simulink model "ROS2_simulink_UE5_0821"  (R2024b)
settings: Solver=VariableStepAuto  StartTime=0.0  StopTime=inf  RelTol=1e-3
undefined symbols (not defined in the file): Aw_pont, B_pont, Cb_pont, dt, Earth, I_L, I_T, IC, Ig_CG, k_neg, k_pos, L, l1, l2, LCF, m, rg, Sim3dSensor, T_yaw, trim_setpoint, Umax, WGS84, x, y, z
libraries: sim3dlib x12, ros2lib x8, matrix_library x8, sharedutil x7, uavsimlib x6, simulink x4, simulink_extras x4, sharedtransform x3, robotcorelib x1, aerolibtransform2 x1, sim3dcameralib x1, visionsinks x1
(part 2 of 2)

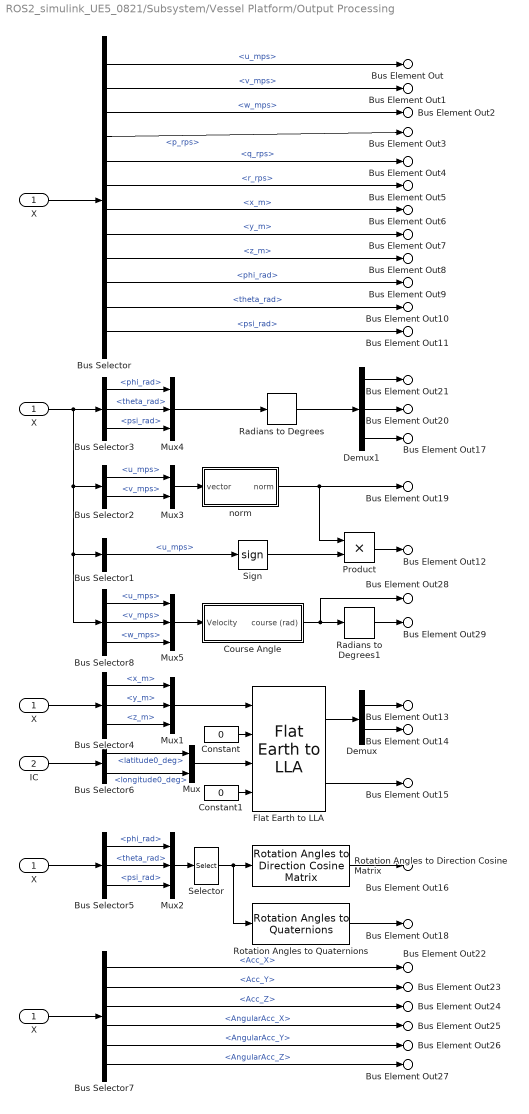
== system ROS2_simulink_UE5_0821/Subsystem/Vessel Platform/Output Processing ==
  X : Inport
  IC : Inport  Port=2
  " X" : InportShadow
  " X  " : InportShadow
  Bus Selector : BusSelector  OutputSignals=u_mps,v_mps,w_mps,p_rps,q_rps,r_rps,x_m,y_m,z_m,phi_rad,theta_rad,psi_rad
  Bus Selector1 : BusSelector  OutputSignals=u_mps
  Bus Selector2 : BusSelector  OutputSignals=u_mps,v_mps
  Bus Selector3 : BusSelector  OutputSignals=phi_rad,theta_rad,psi_rad
  Bus Selector4 : BusSelector  OutputSignals=x_m,y_m,z_m
  Bus Selector5 : BusSelector  OutputSignals=phi_rad,theta_rad,psi_rad
  Bus Selector6 : BusSelector  OutputSignals=latitude0_deg,longitude0_deg
  Bus Selector7 : BusSelector  OutputSignals=Acc_X,Acc_Y,Acc_Z,AngularAcc_X,AngularAcc_Y,AngularAcc_Z
  Bus Selector8 : BusSelector  OutputSignals=u_mps,v_mps,w_mps
  Constant : Constant  Value=0
  Constant1 : Constant  Value=0
  Course Angle : Subsystem
  Demux : Demux  Outputs=2
  Demux1 : Demux  Outputs=3
  Flat Earth to LLA : aerolibtransform2/Flat Earth to LLA  units=Metric (MKS)  ptype=Earth (WGS84)  F=1/298.257223563  R=6378137  refPosPort=on  LL0=ll0  psi=0
  Mux : Mux  Inputs=2
  Mux{1..2,4..5} (4 alike) : Mux  Inputs=3
  Mux3 : Mux  Inputs=2
  Product : Product
  Radians to Degrees : simulink_extras/Transformations/Radians to Degrees
  Radians to Degrees1 : simulink_extras/Transformations/Radians to Degrees
  Rotation Angles to Direction Cosine Matrix : sharedtransform/Rotation Angles to Direction Cosine Matrix  rotationOrder=ZYX  aMode=aMode
  Rotation Angles to Quaternions : sharedtransform/Rotation Angles to Quaternions  rotationOrder=ZYX  aMode=aMode
  Selector : Selector  InputPortWidth=3  IndexOptions=Index vector (dialog)  Indices=[3 2 1]  OutputSizes=1
  Sign : Signum
  "X " : InportShadow
  "X  " : InportShadow
  norm : Subsystem
  Bus Element Out : Outport  PortName=VesselStates  Element=Surge Velocity (m/s)
  Bus Element Out1 : Outport  PortName=VesselStates  Element=Sway Velocity (m/s)
  Bus Element Out2 : Outport  PortName=VesselStates  Element=Heave Velocity (m/s)
  Bus Element Out3 : Outport  PortName=VesselStates  Element=Roll Rate (rad/s)
  Bus Element Out4 : Outport  PortName=VesselStates  Element=Pitch Rate (rad/s)
  Bus Element Out5 : Outport  PortName=VesselStates  Element=Yaw Rate (rad/s)
  Bus Element Out6 : Outport  PortName=VesselStates  Element=x (m)
  Bus Element Out7 : Outport  PortName=VesselStates  Element=y (m)
  Bus Element Out8 : Outport  PortName=VesselStates  Element=z (m)
  Bus Element Out9 : Outport  PortName=VesselStates  Element=Roll Angle (rad)
  Bus Element Out10 : Outport  PortName=VesselStates  Element=Pitch Angle (rad)
  Bus Element Out11 : Outport  PortName=VesselStates  Element=Yaw Angle (rad)
  Bus Element Out21 : Outport  PortName=VesselStates  Element=Roll Angle (deg)
  Bus Element Out20 : Outport  PortName=VesselStates  Element=Pitch Angle (deg)
  Bus Element Out17 : Outport  PortName=VesselStates  Element=Yaw Angle (deg)
  Bus Element Out12 : Outport  PortName=VesselStates  Element=speed (signed m/s)
  Bus Element Out19 : Outport  PortName=VesselStates  Element=speed (unsigned m/s)
  Bus Element Out13 : Outport  PortName=VesselStates  Element=latitude (deg)
  Bus Element Out14 : Outport  PortName=VesselStates  Element=longitude (deg)
  Bus Element Out15 : Outport  PortName=VesselStates  Element=altitude (m)
  Bus Element Out16 : Outport  PortName=VesselStates  Element=DCM_be
  Bus Element Out18 : Outport  PortName=VesselStates  Element=Quaternion
  Bus Element Out22 : Outport  PortName=VesselStates  Element=Acc X (m/s2)
  Bus Element Out23 : Outport  PortName=VesselStates  Element=Acc Y (m/s2)
  Bus Element Out24 : Outport  PortName=VesselStates  Element=Acc Z (m/s2)
  Bus Element Out25 : Outport  PortName=VesselStates  Element=Angular Acc X (rad/s2)
  Bus Element Out26 : Outport  PortName=VesselStates  Element=Angular Acc Y (rad/s2)
  Bus Element Out27 : Outport  PortName=VesselStates  Element=Angular Acc Z (rad/s2)
  Bus Element Out28 : Outport  PortName=VesselStates  Element=course (rad)
  Bus Element Out29 : Outport  PortName=VesselStates  Element=course (deg)
  wires:
  Demux/1 -> Bus Element Out13/1
  Rotation Angles to Quaternions/1 -> Bus Element Out18/1
  Product/1 -> Bus Element Out12/1
  Rotation Angles to Direction Cosine Matrix/1 -> Bus Element Out16/1
  Demux/2 -> Bus Element Out14/1
  Constant/1 -> Flat Earth to LLA/2
  Mux1/1 -> Flat Earth to LLA/1
  Flat Earth to LLA/1 -> Demux/1
  Flat Earth to LLA/2 -> Bus Element Out15/1
  X/1 -> Bus Selector/1
  Bus Selector/1 -> Bus Element Out/1  "<u_mps>"
  Bus Selector/2 -> Bus Element Out1/1  "<v_mps>"
  Bus Selector/3 -> Bus Element Out2/1  "<w_mps>"
  Bus Selector/4 -> Bus Element Out3/1  "<p_rps>"
  Bus Selector/5 -> Bus Element Out4/1  "<q_rps>"
  Bus Selector/6 -> Bus Element Out5/1  "<r_rps>"
  Bus Selector/7 -> Bus Element Out6/1  "<x_m>"
  Bus Selector/8 -> Bus Element Out7/1  "<y_m>"
  Bus Selector/9 -> Bus Element Out8/1  "<z_m>"
  Bus Selector/10 -> Bus Element Out9/1  "<phi_rad>"
  Bus Selector/11 -> Bus Element Out10/1  "<theta_rad>"
  Bus Selector/12 -> Bus Element Out11/1  "<psi_rad>"
  Bus Selector1/1 -> Sign/1  "<u_mps>"
  "X "/1 -> Bus Selector8/1, Bus Selector1/1, Bus Selector2/1, Bus Selector3/1
  Mux3/1 -> norm/1(vector)
  Bus Selector2/1 -> Mux3/1  "<u_mps>"
  Bus Selector2/2 -> Mux3/2  "<v_mps>"
  norm/1(norm) -> Product/1, Bus Element Out19/1
  Bus Selector4/1 -> Mux1/1  "<x_m>"
  Bus Selector4/2 -> Mux1/2  "<y_m>"
  Bus Selector4/3 -> Mux1/3  "<z_m>"
  IC/1 -> Bus Selector6/1
  Bus Selector6/1 -> Mux/1  "<latitude0_deg>"
  Bus Selector6/2 -> Mux/2  "<longitude0_deg>"
  Mux/1 -> Flat Earth to LLA/3
  Selector/1 -> Rotation Angles to Quaternions/1, Rotation Angles to Direction Cosine Matrix/1
  Bus Selector5/1 -> Mux2/1  "<phi_rad>"
  Bus Selector5/2 -> Mux2/2  "<theta_rad>"
  Bus Selector5/3 -> Mux2/3  "<psi_rad>"
  Mux2/1 -> Selector/1
  "X  "/1 -> Bus Selector4/1
  " X"/1 -> Bus Selector5/1
  Bus Selector3/1 -> Mux4/1  "<phi_rad>"
  Bus Selector3/2 -> Mux4/2  "<theta_rad>"
  Bus Selector3/3 -> Mux4/3  "<psi_rad>"
  Mux4/1 -> Radians to Degrees/1
  Radians to Degrees/1 -> Demux1/1
  Demux1/3 -> Bus Element Out17/1
  Demux1/2 -> Bus Element Out20/1
  Demux1/1 -> Bus Element Out21/1
  " X  "/1 -> Bus Selector7/1
  Bus Selector7/1 -> Bus Element Out22/1  "<Acc_X>"
  Bus Selector7/2 -> Bus Element Out23/1  "<Acc_Y>"
  Bus Selector7/3 -> Bus Element Out24/1  "<Acc_Z>"
  Bus Selector7/4 -> Bus Element Out25/1  "<AngularAcc_X>"
  Bus Selector7/5 -> Bus Element Out26/1  "<AngularAcc_Y>"
  Bus Selector7/6 -> Bus Element Out27/1  "<AngularAcc_Z>"
  Constant1/1 -> Flat Earth to LLA/4
  Sign/1 -> Product/2
  Bus Selector8/3 -> Mux5/3  "<w_mps>"
  Bus Selector8/2 -> Mux5/2  "<v_mps>"
  Bus Selector8/1 -> Mux5/1  "<u_mps>"
  Mux5/1 -> Course Angle/1(Velocity)
  Course Angle/1(course (rad)) -> Bus Element Out28/1, Radians to Degrees1/1
  Radians to Degrees1/1 -> Bus Element Out29/1

== system ROS2_simulink_UE5_0821/Subsystem/Vessel Platform/Sum of Forces and Moments ==
  Thrust : Inport
  Crossflow : Inport  Port=2
  Bus Element In7 : Inport  Port=3  PortName=Hydrodynamics  Element=Coriolis
  Bus Element In1 : Inport  Port=3  PortName=Hydrodynamics  Element=Damping
  Bus Element In6 : Inport  Port=4  PortName=Hydrostatic  Element=Hydrostatic
  Bus Element In2 : Inport  Port=4  PortName=Hydrostatic  Element=Ballast
  Add : Sum  Inputs=+++---
  Bus Creator : BusCreator  Inputs=1
  Forces and Moments : Outport
  wires:
  Crossflow/1 -> Add/3
  Bus Element In1/1 -> Add/2
  Bus Element In7/1 -> Add/4
  Thrust/1 -> Add/1
  Add/1 -> Bus Creator/1  "force_moment"
  Bus Creator/1 -> Forces and Moments/1
  Bus Element In6/1 -> Add/5
  Bus Element In2/1 -> Add/6

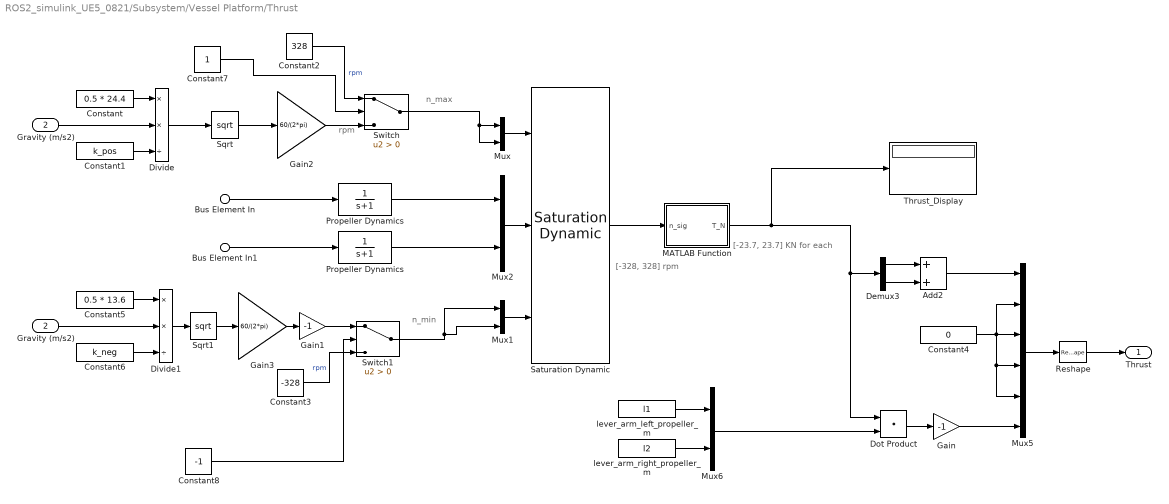
== system ROS2_simulink_UE5_0821/Subsystem/Vessel Platform/Thrust ==
  note: rpm
  note: n_max
  note: n_min
  note: [-23.7, 23.7] KN for each
  note: [-328, 328] rpm
  Bus Element In : Inport  PortName=VesselCmds  Element=PropellerCommand_L_rpm
  Bus Element In1 : Inport  PortName=VesselCmds  Element=PropellerCommand_R_rpm
  "Gravity (m/s2) " : Inport  Port=2
  Add2 : Sum
  Constant : Constant  Value=0.5 * 24.4
  Constant1 : Constant  Value=k_pos
  Constant2 : Constant  Value=328
  Constant3 : Constant  Value=-328
  Constant4 : Constant  Value=0
  Constant5 : Constant  Value=0.5 * 13.6
  Constant6 : Constant  Value=k_neg
  Constant7 : Constant
  Constant8 : Constant  Value=-1
  Demux3 : Demux  Outputs=2
  Divide : Product  Inputs=**/
  Divide1 : Product  Inputs=**/
  Dot Product : DotProduct  OutDataTypeStr=Inherit: Inherit via internal rule
  Gain : Gain  Gain=-1
  Gain1 : Gain  Gain=-1
  Gain2 : Gain  Gain=60/(2*pi)
  Gain3 : Gain  Gain=60/(2*pi)
  "Gravity (m/s2)  " : InportShadow  Port=2
  MATLAB Function : MATLAB Function  TreatAsAtomicUnit=on
  Mux{,1..2,6} (4 alike) : Mux  Inputs=2
  Mux5 : Mux  Inputs=6
  Propeller Dynamics : TransferFcn  Denominator=[1 1]
  "Propeller Dynamics " : TransferFcn  Denominator=[1 1]
  Reshape : Reshape  OutputDimensionality=Column vector (2-D)
  Saturation Dynamic : simulink/Discontinuities/Saturation Dynamic  OutMin=[]  OutMax=[]  OutDataTypeStr=Inherit: Same as second input  OutDataType=fixdt(1, 16)  OutScaling=2^-10  DoSatur=off
  Sqrt : Sqrt
  Sqrt1 : Sqrt
  Switch : Switch  Criteria=u2 > Threshold  SaturateOnIntegerOverflow=off  InputSameDT=off
  Switch1 : Switch  Criteria=u2 > Threshold  SaturateOnIntegerOverflow=off  InputSameDT=off
  Thrust_Display : Display
  lever_arm_left_propeller_m : Constant  Value=l1
  lever_arm_right_propeller_m : Constant  Value=l2
  Thrust : Outport
  wires:
  Saturation Dynamic/1 -> MATLAB Function/1(n_sig)
  Demux3/2 -> Add2/2
  Dot Product/1 -> Gain/1
  Gain/1 -> Mux5/6
  Mux5/1 -> Reshape/1
  Mux6/1 -> Dot Product/2
  Add2/1 -> Mux5/1
  Constant4/1 -> Mux5/5, Mux5/4, Mux5/2, Mux5/3
  Demux3/1 -> Add2/1
  lever_arm_right_propeller_m/1 -> Mux6/2
  lever_arm_left_propeller_m/1 -> Mux6/1
  Reshape/1 -> Thrust/1
  Constant/1 -> Divide/1
  "Gravity (m/s2) "/1 -> Divide/2
  Constant1/1 -> Divide/3
  Divide/1 -> Sqrt/1
  Divide1/1 -> Sqrt1/1
  Constant5/1 -> Divide1/1
  "Gravity (m/s2)  "/1 -> Divide1/2
  Constant6/1 -> Divide1/3
  Sqrt1/1 -> Gain3/1
  Mux/1 -> Saturation Dynamic/1
  Sqrt/1 -> Gain2/1
  Mux1/1 -> Saturation Dynamic/3
  Mux2/1 -> Saturation Dynamic/2
  Bus Element In/1 -> Propeller Dynamics/1
  Bus Element In1/1 -> "Propeller Dynamics "/1
  "Propeller Dynamics "/1 -> Mux2/2
  Gain2/1 -> Switch/3
  MATLAB Function/1(T_N) -> Thrust_Display/1, Dot Product/1, Demux3/1
  Propeller Dynamics/1 -> Mux2/1
  Switch/1 -> Mux/1, Mux/2
  Constant2/1 -> Switch/1  "rpm"
  Gain3/1 -> Gain1/1
  Gain1/1 -> Switch1/1
  Switch1/1 -> Mux1/2, Mux1/1
  Constant3/1 -> Switch1/3  "rpm"
  Constant7/1 -> Switch/2
  Constant8/1 -> Switch1/2

== system ROS2_simulink_UE5_0821/Subsystem/Vessel Platform/Waves and Crossflow ==
  RelativeVelocity : Inport
  Draft (m) : Inport  Port=2
  "Water Density (kg/m3) " : Inport  Port=3
  Compute tau_crossflow : MATLAB Function  TreatAsAtomicUnit=on
  beam_pontoon_m : Constant  Value=B_pont
  length_m : Constant  Value=L
  Crossflow : Outport
  wires:
  length_m/1 -> Compute tau_crossflow/1(L)
  RelativeVelocity/1 -> Compute tau_crossflow/4(nu_r)
  Compute tau_crossflow/1(tau_crossflow) -> Crossflow/1
  beam_pontoon_m/1 -> Compute tau_crossflow/2(B)
  "Water Density (kg/m3) "/1 -> Compute tau_crossflow/5(rho)
  Draft (m)/1 -> Compute tau_crossflow/3(T)

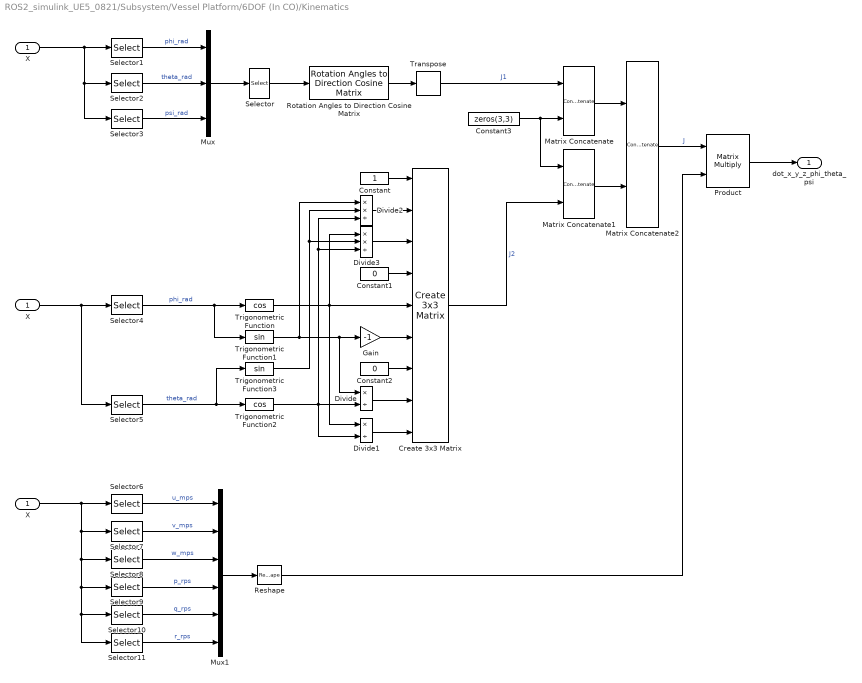
== system ROS2_simulink_UE5_0821/Subsystem/Vessel Platform/6DOF (In CO)/Kinematics ==
  X : Inport
  Constant : Constant
  Constant1 : Constant  Value=0
  Constant2 : Constant  Value=0
  Constant3 : Constant  Value=zeros(3,3)
  Create 3x3 Matrix : sharedutil/Create 3x3 Matrix  aMode=aMode
  Divide : Product  Inputs=*/
  Divide1 : Product  Inputs=*/
  Divide2 : Product  Inputs=**/
  Divide3 : Product  Inputs=**/
  Gain : Gain  Gain=-1
  Matrix Concatenate : Concatenate  Mode=Multidimensional array  ConcatenateDimension=2
  Matrix Concatenate1 : Concatenate  Mode=Multidimensional array  ConcatenateDimension=2
  Matrix Concatenate2 : Concatenate  Mode=Multidimensional array
  Mux : Mux  Inputs=3
  Mux1 : Mux  Inputs=6
  Product : Product  Multiplication=Matrix(*)
  Reshape : Reshape  OutputDimensionality=Column vector (2-D)
  Rotation Angles to Direction Cosine Matrix : sharedtransform/Rotation Angles to Direction Cosine Matrix  rotationOrder=ZYX  aMode=aMode
  Selector : Selector  InputPortWidth=3  IndexOptions=Index vector (dialog)  Indices=[3 2 1]  OutputSizes=1
  Selector1 : Selector  InputPortWidth=12  IndexOptions=Index vector (dialog)  Indices=[10]  OutputSizes=1
  Selector10 : Selector  InputPortWidth=12  IndexOptions=Index vector (dialog)  Indices=[5]  OutputSizes=1
  Selector11 : Selector  InputPortWidth=12  IndexOptions=Index vector (dialog)  Indices=[6]  OutputSizes=1
  Selector2 : Selector  InputPortWidth=12  IndexOptions=Index vector (dialog)  Indices=[11]  OutputSizes=1
  Selector3 : Selector  InputPortWidth=12  IndexOptions=Index vector (dialog)  Indices=[12]  OutputSizes=1
  Selector4 : Selector  InputPortWidth=12  IndexOptions=Index vector (dialog)  Indices=[10]  OutputSizes=1
  Selector5 : Selector  InputPortWidth=12  IndexOptions=Index vector (dialog)  Indices=[11]  OutputSizes=1
  Selector6 : Selector  InputPortWidth=12  IndexOptions=Index vector (dialog)  Indices=[1]  OutputSizes=1
  Selector7 : Selector  InputPortWidth=12  IndexOptions=Index vector (dialog)  Indices=[2]  OutputSizes=1
  Selector8 : Selector  InputPortWidth=12  IndexOptions=Index vector (dialog)  Indices=[3]  OutputSizes=1
  Selector9 : Selector  InputPortWidth=12  IndexOptions=Index vector (dialog)  Indices=[4]  OutputSizes=1
  Transpose : matrix_library/Transpose
  Trigonometric Function : Trigonometry  Operator=cos
  Trigonometric Function1 : Trigonometry
  Trigonometric Function2 : Trigonometry  Operator=cos
  Trigonometric Function3 : Trigonometry
  "X " : InportShadow
  "X  " : InportShadow
  dot_x_y_z_phi_theta_psi : Outport
  wires:
  Rotation Angles to Direction Cosine Matrix/1 -> Transpose/1
  Selector/1 -> Rotation Angles to Direction Cosine Matrix/1
  Selector1/1 -> Mux/1  "phi_rad"
  Selector2/1 -> Mux/2  "theta_rad"
  Selector3/1 -> Mux/3  "psi_rad"
  Mux/1 -> Selector/1
  Constant/1 -> Create 3x3 Matrix/1
  Constant1/1 -> Create 3x3 Matrix/4
  Constant2/1 -> Create 3x3 Matrix/7
  Trigonometric Function/1 -> Divide3/1, Divide1/1, Create 3x3 Matrix/5
  Selector4/1 -> Trigonometric Function1/1, Trigonometric Function/1  "phi_rad"
  Trigonometric Function1/1 -> Divide/1, Gain/1, Divide2/1
  Gain/1 -> Create 3x3 Matrix/6
  Selector5/1 -> Trigonometric Function3/1, Trigonometric Function2/1  "theta_rad"
  Divide/1 -> Create 3x3 Matrix/8
  Trigonometric Function2/1 -> Divide3/3, Divide2/3, Divide1/2, Divide/2
  Divide1/1 -> Create 3x3 Matrix/9
  Divide2/1 -> Create 3x3 Matrix/2
  Divide3/1 -> Create 3x3 Matrix/3
  Trigonometric Function3/1 -> Divide3/2, Divide2/2
  Matrix Concatenate/1 -> Matrix Concatenate2/1
  Matrix Concatenate1/1 -> Matrix Concatenate2/2
  Transpose/1 -> Matrix Concatenate/1  "J1"
  Constant3/1 -> Matrix Concatenate/2, Matrix Concatenate1/1
  Create 3x3 Matrix/1 -> Matrix Concatenate1/2  "J2"
  Selector6/1 -> Mux1/1  "u_mps"
  Selector7/1 -> Mux1/2  "v_mps"
  Selector8/1 -> Mux1/3  "w_mps"
  Selector9/1 -> Mux1/4  "p_rps"
  Selector10/1 -> Mux1/5  "q_rps"
  Selector11/1 -> Mux1/6  "r_rps"
  Mux1/1 -> Reshape/1
  X/1 -> Selector3/1, Selector2/1, Selector1/1
  "X "/1 -> Selector5/1, Selector4/1
  "X  "/1 -> Selector7/1, Selector8/1, Selector9/1, Selector10/1, Selector11/1, Selector6/1
  Matrix Concatenate2/1 -> Product/1  "J"
  Reshape/1 -> Product/2
  Product/1 -> dot_x_y_z_phi_theta_psi/1

== system ROS2_simulink_UE5_0821/Subsystem/Vessel Platform/6DOF (In CO)/ssa    ==
  angle : Inport
  " " : Math  Operator=mod
  Constant : Constant  Value=2*pi
  Constant1 : Constant  Value=pi
  Sum : Sum  Inputs=++|
  Sum1 : Sum  Inputs=-+|
  angle_pipi : Outport
  wires:
  Sum/1 -> " "/1
  Constant1/1 -> Sum/1, Sum1/1
  " "/1 -> Sum1/2
  Sum1/1 -> angle_pipi/1
  Constant/1 -> " "/2
  angle/1 -> Sum/2

== system ROS2_simulink_UE5_0821/Subsystem/Vessel Platform/Hydrodynamics/Coriolis  ==
  Relative Velocity : Inport
  Transform CG to CO : Inport  Port=2
  Inertial Matrix (hull and payload) in CO : Inport  Port=3
  X : Inport  Port=4
  Added Mass (Hydrodynamics) : Inport  Port=5
  Inertials : Inport  Port=6
  Bus Selector : BusSelector  OutputSignals=p_rps,q_rps,r_rps
  Bus Selector1 : BusSelector  OutputSignals=mp
  Compute CA : MATLAB Function  TreatAsAtomicUnit=on
  Comupute CRB : Subsystem
  Mux : Mux  Inputs=3
  Product : Product  Multiplication=Matrix(*)
  "Relative Velocity " : InportShadow
  Reshape : Reshape  OutputDimensionality=Column vector (2-D)
  Sum : Sum  Inputs=+|+
  Coriolis : Outport
  wires:
  Comupute CRB/1(CRB) -> Sum/2  "CRB"
  Added Mass (Hydrodynamics)/1 -> Compute CA/1(MA)
  "Relative Velocity "/1 -> Reshape/1
  Sum/1 -> Product/1  "C"
  Compute CA/1(CA) -> Sum/1  "CA"
  Reshape/1 -> Product/2
  Product/1 -> Coriolis/1
  Relative Velocity/1 -> Compute CA/2(nu_r)
  Bus Selector/1 -> Mux/1  "<p_rps>"
  Bus Selector/2 -> Mux/2  "<q_rps>"
  Bus Selector/3 -> Mux/3  "<r_rps>"
  Mux/1 -> Comupute CRB/1(pqr)
  X/1 -> Bus Selector/1
  Transform CG to CO/1 -> Comupute CRB/2(H)
  Inertial Matrix (hull and payload) in CO/1 -> Comupute CRB/3(Ig)
  Inertials/1 -> Bus Selector1/1
  Bus Selector1/1 -> Comupute CRB/4(mp)  "<mp>"

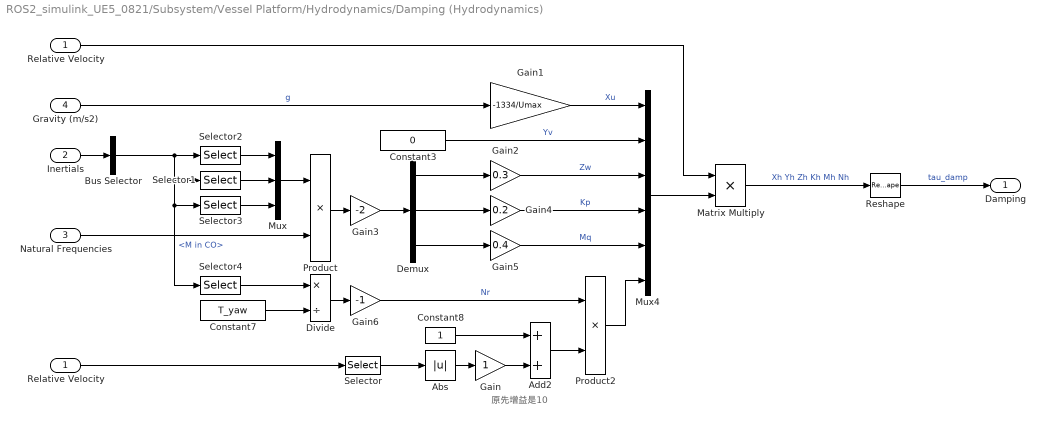
== system ROS2_simulink_UE5_0821/Subsystem/Vessel Platform/Hydrodynamics/Damping (Hydrodynamics) ==
  note: 原先增益是10
  Relative Velocity : Inport
  Inertials : Inport  Port=2
  Natural Frequencies : Inport  Port=3
  "Gravity (m/s2) " : Inport  Port=4
  Abs : Abs  SaturateOnIntegerOverflow=off
  Add2 : Sum
  Bus Selector : BusSelector  OutputSignals=M in CO
  Constant3 : Constant  Value=0
  Constant7 : Constant  Value=T_yaw
  Constant8 : Constant
  Demux : Demux  Outputs=3
  Divide : Product  Inputs=*/
  Gain : Gain
  Gain1 : Gain  Gain=-1334/Umax
  Gain2 : Gain  Gain=0.3
  Gain3 : Gain  Gain=-2
  Gain4 : Gain  Gain=0.2
  Gain5 : Gain  Gain=0.4
  Gain6 : Gain  Gain=-1
  Matrix Multiply : Product
  Mux : Mux  Inputs=3
  Mux4 : Mux  Inputs=6
  Product : Product
  Product2 : Product
  "Relative Velocity " : InportShadow
  Reshape : Reshape  OutputDimensionality=Column vector (2-D)
  Selector : Selector  InputPortWidth=6  IndexOptions=Index vector (dialog)  Indices=[6]  OutputSizes=1
  Selector1 : Selector  NumberOfDimensions=2  InputPortWidth=3  IndexOptions=Index vector (dialog),Index vector (dialog)  Indices=4,4  OutputSizes=1,1
  Selector2 : Selector  NumberOfDimensions=2  InputPortWidth=3  IndexOptions=Index vector (dialog),Index vector (dialog)  Indices=3,3  OutputSizes=1,1
  Selector3 : Selector  NumberOfDimensions=2  InputPortWidth=3  IndexOptions=Index vector (dialog),Index vector (dialog)  Indices=5,5  OutputSizes=1,1
  Selector4 : Selector  NumberOfDimensions=2  InputPortWidth=3  IndexOptions=Index vector (dialog),Index vector (dialog)  Indices=6,6  OutputSizes=1,1
  Damping : Outport
  wires:
  Constant3/1 -> Mux4/2  "Yv"
  Gain/1 -> Add2/2
  Gain1/1 -> Mux4/1  "Xu"
  Constant8/1 -> Add2/1
  Selector/1 -> Abs/1
  Demux/2 -> Gain4/1
  Gain6/1 -> Product2/1  "Nr"
  Product2/1 -> Mux4/6
  Abs/1 -> Gain/1
  Gain5/1 -> Mux4/5  "Mq"
  Gain2/1 -> Mux4/3  "Zw"
  Add2/1 -> Product2/2
  Mux4/1 -> Matrix Multiply/2
  Relative Velocity/1 -> Matrix Multiply/1
  Matrix Multiply/1 -> Reshape/1  "Xh Yh Zh Kh Mh Nh"
  Reshape/1 -> Damping/1  "tau_damp"
  "Gravity (m/s2) "/1 -> Gain1/1  "g"
  "Relative Velocity "/1 -> Selector/1
  Inertials/1 -> Bus Selector/1
  Bus Selector/1 -> Selector1/1, Selector4/1, Selector3/1, Selector2/1  "<M in CO>"
  Selector2/1 -> Mux/1
  Selector1/1 -> Mux/2
  Selector3/1 -> Mux/3
  Mux/1 -> Product/1
  Natural Frequencies/1 -> Product/2
  Product/1 -> Gain3/1
  Demux/1 -> Gain2/1
  Gain3/1 -> Demux/1
  Gain4/1 -> Mux4/4  "Kp"
  Demux/3 -> Gain5/1
  Selector4/1 -> Divide/1
  Constant7/1 -> Divide/2
  Divide/1 -> Gain6/1

== system ROS2_simulink_UE5_0821/Subsystem/Vessel Platform/Hydrostatic/Ballast ==
  Constant : Constant  Value=0
  Constant9 : Constant  Value=trim_setpoint
  Mux : Mux  Inputs=6
  Reshape : Reshape  OutputDimensionality=Column vector (2-D)
  Transfer Fcn2 : TransferFcn  Denominator=[1 1]
  Ballast : Outport
  wires:
  Constant9/1 -> Transfer Fcn2/1
  Transfer Fcn2/1 -> Mux/5
  Constant/1 -> Mux/2, Mux/3, Mux/6, Mux/4, Mux/1
  Mux/1 -> Reshape/1
  Reshape/1 -> Ballast/1

== system ROS2_simulink_UE5_0821/Subsystem/Vessel Platform/Input Processing/Added Mass (Hydrodynamics)  ==
  Inertial Matrix (hull and payload) in CO : Inport
  Create Diagonal Matrix : matrix_library/Create Diagonal Matrix
  Gain : Gain  Gain=-0.1
  Gain1 : Gain  Gain=-1
  Gain2 : Gain  Gain=-1.5
  Gain3 : Gain  Gain=-1
  Gain4 : Gain  Gain=-0.2
  Gain5 : Gain  Gain=-0.8
  Gain6 : Gain  Gain=-1.7
  Mux : Mux  Inputs=6
  Selector : Selector  NumberOfDimensions=2  InputPortWidth=3  IndexOptions=Index vector (dialog),Index vector (dialog)  Indices=1,1  OutputSizes=1,1
  Selector1 : Selector  NumberOfDimensions=2  InputPortWidth=3  IndexOptions=Index vector (dialog),Index vector (dialog)  Indices=2,2  OutputSizes=1,1
  Selector2 : Selector  NumberOfDimensions=2  InputPortWidth=3  IndexOptions=Index vector (dialog),Index vector (dialog)  Indices=3,3  OutputSizes=1,1
  "mass (kg) " : Constant  Value=m
  Added Mass (Hydrodynamcis) : Outport
  wires:
  Gain1/1 -> Added Mass (Hydrodynamcis)/1
  "mass (kg) "/1 -> Gain3/1, Gain2/1, Gain/1
  Create Diagonal Matrix/1 -> Gain1/1
  Mux/1 -> Create Diagonal Matrix/1
  Gain/1 -> Mux/1  "Xudot"
  Gain2/1 -> Mux/2  "Yvdot"
  Gain3/1 -> Mux/3  "Zwdot"
  Gain4/1 -> Mux/4  "Kpdot"
  Gain5/1 -> Mux/5  "Mqdot"
  Gain6/1 -> Mux/6  "Nrdot"
  Inertial Matrix (hull and payload) in CO/1 -> Selector2/1, Selector1/1, Selector/1  "Ig"
  Selector/1 -> Gain4/1
  Selector1/1 -> Gain5/1
  Selector2/1 -> Gain6/1

== system ROS2_simulink_UE5_0821/Subsystem/Vessel Platform/Input Processing/CG corrected for payload ==
  mp : Inport
  rp : Inport  Port=2
  Add1 : Sum
  Add2 : Sum
  CG hull only (m) : Constant  Value=rg
  Divide1 : Product  Inputs=*/
  Product : Product
  Product1 : Product
  "mass (kg) " : Constant  Value=m
  CG corrected for payload (m) : Outport
  wires:
  Add2/1 -> Divide1/2
  "mass (kg) "/1 -> Add2/1, Product/1
  mp/1 -> Add2/2, Product1/1
  CG hull only (m)/1 -> Product/2
  Product/1 -> Add1/1
  Product1/1 -> Add1/2
  Add1/1 -> Divide1/1
  rp/1 -> Product1/2
  Divide1/1 -> CG corrected for payload (m)/1  "rg"

== system ROS2_simulink_UE5_0821/Subsystem/Vessel Platform/Input Processing/Draft (m)  ==
  nabla : Inport
  Constant6 : Constant  Value=2
  Divide7 : Product  Inputs=*////
  "beam pontoon (m)  " : Constant  Value=B_pont
  block coefficient : Constant  Value=Cb_pont
  "length (m) " : Constant  Value=L
  T : Outport
  wires:
  "length (m) "/1 -> Divide7/5
  "beam pontoon (m)  "/1 -> Divide7/4
  Constant6/1 -> Divide7/2
  Divide7/1 -> T/1  "draft"
  block coefficient/1 -> Divide7/3
  nabla/1 -> Divide7/1

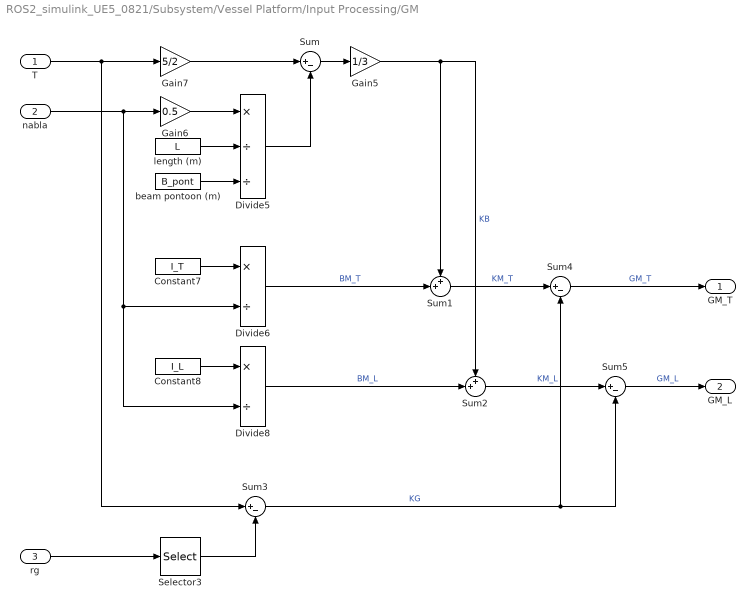
== system ROS2_simulink_UE5_0821/Subsystem/Vessel Platform/Input Processing/GM ==
  T : Inport
  nabla : Inport  Port=2
  rg : Inport  Port=3
  Constant7 : Constant  Value=I_T
  Constant8 : Constant  Value=I_L
  Divide5 : Product  Inputs=*//
  Divide6 : Product  Inputs=*/
  Divide8 : Product  Inputs=*/
  Gain5 : Gain  Gain=1/3
  Gain6 : Gain  Gain=0.5
  Gain7 : Gain  Gain=5/2
  Selector3 : Selector  InputPortWidth=3  IndexOptions=Index vector (dialog)  Indices=3  OutputSizes=1
  Sum{,3..5} (4 alike) : Sum  Inputs=|+-
  Sum1 : Sum  Inputs=++|
  Sum2 : Sum  Inputs=++|
  beam pontoon (m) : Constant  Value=B_pont
  length (m) : Constant  Value=L
  GM_T : Outport
  GM_L : Outport  Port=2
  wires:
  Divide6/1 -> Sum1/2  "BM_T"
  Sum3/1 -> Sum5/2, Sum4/2  "KG"
  Gain7/1 -> Sum/1
  Gain6/1 -> Divide5/1
  Gain5/1 -> Sum2/1, Sum1/1  "KB"
  T/1 -> Gain7/1, Sum3/1
  Constant8/1 -> Divide8/1
  beam pontoon (m)/1 -> Divide5/3
  nabla/1 -> Divide8/2, Divide6/2, Gain6/1
  length (m)/1 -> Divide5/2
  Sum/1 -> Gain5/1
  Constant7/1 -> Divide6/1
  Divide5/1 -> Sum/2
  Divide8/1 -> Sum2/2  "BM_L"
  Selector3/1 -> Sum3/2
  Sum2/1 -> Sum5/1  "KM_L"
  Sum1/1 -> Sum4/1  "KM_T"
  Sum5/1 -> GM_L/1  "GM_L"
  Sum4/1 -> GM_T/1  "GM_T"
  rg/1 -> Selector3/1

== system ROS2_simulink_UE5_0821/Subsystem/Vessel Platform/Input Processing/G_CF (spring stiffness matrix in the CF) ==
  rho : Inport
  g : Inport  Port=2
  nabla : Inport  Port=3
  GM_T : Inport  Port=4
  GM_L : Inport  Port=5
  Constant : Constant  Value=0
  Create Diagonal Matrix : matrix_library/Create Diagonal Matrix
  Gain2 : Gain  Gain=2 * Aw_pont
  Mux : Mux  Inputs=6
  Product{6..7,9..10} (4 alike) : Product
  G_CF : Outport
  G33 : Outport  Port=2
  G44 : Outport  Port=3
  G55 : Outport  Port=4
  wires:
  Gain2/1 -> G33/1, Mux/3
  Mux/1 -> Create Diagonal Matrix/1
  Product7/1 -> Product9/1, Product10/1
  Product10/1 -> G55/1, Mux/5
  Product9/1 -> G44/1, Mux/4
  GM_T/1 -> Product9/2
  Constant/1 -> Mux/6, Mux/2, Mux/1
  Product6/1 -> Product7/1, Gain2/1
  GM_L/1 -> Product10/2
  g/1 -> Product6/2
  rho/1 -> Product6/1
  nabla/1 -> Product7/2
  Create Diagonal Matrix/1 -> G_CF/1  "G_CF (spring stiffness matrix in the CF)"

== system ROS2_simulink_UE5_0821/Subsystem/Vessel Platform/Input Processing/Inertial Matrix (hull and payload) in CO  ==
  rp : Inport
  mp : Inport  Port=2
  Add3 : Sum  Inputs=+--
  "CG hull only (m) " : Constant  Value=rg
  Gain : Gain  Gain=m
  Inertial Matrix in CG : Constant  Value=Ig_CG
  Product11 : Product
  Product2 : Product  Multiplication=Matrix(*)
  Product3 : Product  Multiplication=Matrix(*)
  Smtrx : Subsystem
  Smtrx1 : Subsystem
  Ig : Outport
  wires:
  "CG hull only (m) "/1 -> Smtrx/1(a)
  Smtrx1/1(S) -> Product3/2, Product3/1
  mp/1 -> Product11/2
  Gain/1 -> Add3/2
  Smtrx/1(S) -> Product2/2, Product2/1
  Product2/1 -> Gain/1
  Inertial Matrix in CG/1 -> Add3/1
  Product3/1 -> Product11/1
  Product11/1 -> Add3/3
  rp/1 -> Smtrx1/1(a)
  Add3/1 -> Ig/1  "Ig"

== system ROS2_simulink_UE5_0821/Subsystem/Vessel Platform/Input Processing/MRB_CG ==
  mp : Inport
  Ig : Inport  Port=2
  " mass (kg)" : Constant  Value=m
  Add4 : Sum
  Constant1 : Constant  Value=zeros(3,3)
  Constant2 : Constant  Value=eye(3)
  Matrix Concatenate : Concatenate  Mode=Multidimensional array  ConcatenateDimension=2
  Matrix Concatenate1 : Concatenate  Mode=Multidimensional array  ConcatenateDimension=2
  Matrix Concatenate2 : Concatenate  Mode=Multidimensional array
  Product4 : Product
  MRB_CG : Outport
  wires:
  Add4/1 -> Product4/1
  Constant1/1 -> Matrix Concatenate1/1, Matrix Concatenate/2
  Constant2/1 -> Product4/2
  Matrix Concatenate/1 -> Matrix Concatenate2/1
  Product4/1 -> Matrix Concatenate/1
  Matrix Concatenate1/1 -> Matrix Concatenate2/2
  " mass (kg)"/1 -> Add4/1
  mp/1 -> Add4/2
  Matrix Concatenate2/1 -> MRB_CG/1  "MRB_CG"
  Ig/1 -> Matrix Concatenate1/2

== system ROS2_simulink_UE5_0821/Subsystem/Vessel Platform/Input Processing/Natural Frequencies  ==
  G33 : Inport
  G44 : Inport  Port=2
  G55 : Inport  Port=3
  M : Inport  Port=4
  Divide2 : Product  Inputs=*/
  Divide3 : Product  Inputs=*/
  Divide4 : Product  Inputs=*/
  Mux2 : Mux  Inputs=3
  Selector : Selector  NumberOfDimensions=2  InputPortWidth=3  IndexOptions=Index vector (dialog),Index vector (dialog)  Indices=3,3  OutputSizes=1,1
  Selector1 : Selector  NumberOfDimensions=2  InputPortWidth=3  IndexOptions=Index vector (dialog),Index vector (dialog)  Indices=4,4  OutputSizes=1,1
  Selector2 : Selector  NumberOfDimensions=2  InputPortWidth=3  IndexOptions=Index vector (dialog),Index vector (dialog)  Indices=5,5  OutputSizes=1,1
  Sqrt : Sqrt
  w3 w4 w5 : Outport
  wires:
  Selector2/1 -> Divide4/2
  Selector1/1 -> Divide3/2
  Divide3/1 -> Mux2/2
  Mux2/1 -> Sqrt/1
  Divide2/1 -> Mux2/1
  Sqrt/1 -> w3 w4 w5/1  "w3 w4 w5"
  Selector/1 -> Divide2/2
  Divide4/1 -> Mux2/3
  G55/1 -> Divide4/1
  M/1 -> Selector1/1, Selector2/1, Selector/1
  G44/1 -> Divide3/1
  G33/1 -> Divide2/1

== system ROS2_simulink_UE5_0821/Subsystem/Vessel Platform/Input Processing/Relative Velocity  ==
  V_c : Inport
  beta_c : Inport  Port=2
  X : Inport  Port=3
  Add : Sum  Inputs=+-
  Add1 : Sum  Inputs=+-
  Bus Selector : BusSelector  OutputSignals=psi_rad
  Bus Selector1 : BusSelector  OutputSignals=u_mps,v_mps,w_mps,p_rps,q_rps,r_rps
  Constant : Constant  Value=[0 0 0 0]'
  Mux : Mux  Inputs=6
  Mux3 : Mux  Inputs=3
  Product : Product
  Product1 : Product
  Trigonometric Function : Trigonometry  Operator=cos
  Trigonometric Function1 : Trigonometry
  X1 : InportShadow  Port=3
  Relative Velocity : Outport
  wires:
  Product1/1 -> Mux3/2  "v_c_mps"
  V_c/1 -> Product1/2, Product/2
  Trigonometric Function1/1 -> Product1/1
  beta_c/1 -> Add/1
  Add/1 -> Trigonometric Function1/1, Trigonometric Function/1
  Trigonometric Function/1 -> Product/1
  Product/1 -> Mux3/1  "u_c_mps"
  Constant/1 -> Mux3/3
  X/1 -> Bus Selector/1
  Bus Selector/1 -> Add/2  "<psi_rad>"
  X1/1 -> Bus Selector1/1
  Bus Selector1/1 -> Mux/1  "<u_mps>"
  Bus Selector1/2 -> Mux/2  "<v_mps>"
  Bus Selector1/3 -> Mux/3  "<w_mps>"
  Bus Selector1/4 -> Mux/4  "<p_rps>"
  Bus Selector1/5 -> Mux/5  "<q_rps>"
  Bus Selector1/6 -> Mux/6  "<r_rps>"
  Mux3/1 -> Add1/2
  Mux/1 -> Add1/1
  Add1/1 -> Relative Velocity/1

== system ROS2_simulink_UE5_0821/Subsystem/Vessel Platform/Input Processing/Transform CF to CO ==
  r : Inport
  Constant1 : Constant  Value=zeros(3,3)
  Constant2 : Constant  Value=eye(3)
  Constant3 : Constant  Value=eye(3)
  Matrix Concatenate : Concatenate  Mode=Multidimensional array  ConcatenateDimension=2
  Matrix Concatenate1 : Concatenate  Mode=Multidimensional array  ConcatenateDimension=2
  Matrix Concatenate2 : Concatenate  Mode=Multidimensional array
  Smtrx : Subsystem
  Transpose : matrix_library/Transpose
  H : Outport
  wires:
  r/1 -> Smtrx/1(a)
  Constant1/1 -> Matrix Concatenate1/1
  Constant2/1 -> Matrix Concatenate/1
  Matrix Concatenate1/1 -> Matrix Concatenate2/2
  Matrix Concatenate/1 -> Matrix Concatenate2/1
  Constant3/1 -> Matrix Concatenate1/2
  Smtrx/1(S) -> Transpose/1
  Transpose/1 -> Matrix Concatenate/2
  Matrix Concatenate2/1 -> H/1

== system ROS2_simulink_UE5_0821/Subsystem/Vessel Platform/Input Processing/Transform CG to CO  ==
  r : Inport
  Constant1 : Constant  Value=zeros(3,3)
  Constant2 : Constant  Value=eye(3)
  Constant3 : Constant  Value=eye(3)
  Matrix Concatenate : Concatenate  Mode=Multidimensional array  ConcatenateDimension=2
  Matrix Concatenate1 : Concatenate  Mode=Multidimensional array  ConcatenateDimension=2
  Matrix Concatenate2 : Concatenate  Mode=Multidimensional array
  Smtrx : Subsystem
  Transpose : matrix_library/Transpose
  H : Outport
  wires:
  r/1 -> Smtrx/1(a)
  Constant1/1 -> Matrix Concatenate1/1
  Constant2/1 -> Matrix Concatenate/1
  Matrix Concatenate1/1 -> Matrix Concatenate2/2
  Matrix Concatenate/1 -> Matrix Concatenate2/1
  Constant3/1 -> Matrix Concatenate1/2
  Smtrx/1(S) -> Transpose/1
  Transpose/1 -> Matrix Concatenate/2
  Matrix Concatenate2/1 -> H/1

== system ROS2_simulink_UE5_0821/Subsystem/Vessel Platform/Input Processing/Volume ==
  mp : Inport
  rho : Inport  Port=2
  Add : Sum
  Divide : Product  Inputs=*/
  mass (kg) : Constant  Value=m
  Volume (m3) : Outport
  wires:
  mass (kg)/1 -> Add/1
  Add/1 -> Divide/1
  Divide/1 -> Volume (m3)/1  "Volume (m3)"
  rho/1 -> Divide/2
  mp/1 -> Add/2

== system ROS2_simulink_UE5_0821/Subsystem/Vessel Platform/Output Processing/Course Angle ==
  Velocity : Inport
  Atan1 : Trigonometry  Operator=atan2
  Selector : Selector  InputPortWidth=3  IndexOptions=Index vector (dialog)  Indices=[2]  OutputSizes=1
  Selector1 : Selector  InputPortWidth=3  IndexOptions=Index vector (dialog)  Indices=[1]  OutputSizes=1
  course (rad) : Outport
  wires:
  Velocity/1 -> Selector1/1, Selector/1
  Selector1/1 -> Atan1/2
  Selector/1 -> Atan1/1
  Atan1/1 -> course (rad)/1

== system ROS2_simulink_UE5_0821/Subsystem/Vessel Platform/Output Processing/norm ==
  vector : Inport
  Dot Product : DotProduct  OutDataTypeStr=Inherit: Inherit via internal rule
  Sqrt : Sqrt
  norm : Outport
  wires:
  vector/1 -> Dot Product/2, Dot Product/1
  Dot Product/1 -> Sqrt/1
  Sqrt/1 -> norm/1

== system ROS2_simulink_UE5_0821/Subsystem/Vessel Platform/Hydrodynamics/Coriolis /Comupute CRB ==
  pqr : Inport
  H : Inport  Port=2
  Ig : Inport  Port=3
  mp : Inport  Port=4
  " mass (kg) " : Constant  Value=m
  Constant1 : Constant  Value=zeros(3,3)
  Gain1 : Gain  Gain=-1
  Matrix Concatenate : Concatenate  Mode=Multidimensional array  ConcatenateDimension=2
  Matrix Concatenate1 : Concatenate  Mode=Multidimensional array  ConcatenateDimension=2
  Matrix Concatenate2 : Concatenate  Mode=Multidimensional array
  Product : Product  Inputs=3  Multiplication=Matrix(*)
  Product1 : Product
  Product2 : Product  Multiplication=Matrix(*)
  Smtrx : Subsystem
  "Smtrx " : Subsystem
  Sum : Sum  Inputs=++|
  Transpose : matrix_library/Transpose
  CRB : Outport
  wires:
  Matrix Concatenate1/1 -> Matrix Concatenate2/2
  Constant1/1 -> Matrix Concatenate1/1, Matrix Concatenate/2
  Product2/1 -> "Smtrx "/1(a)
  Gain1/1 -> Matrix Concatenate1/2
  Matrix Concatenate/1 -> Matrix Concatenate2/1
  Matrix Concatenate2/1 -> Product/2
  Product/1 -> CRB/1
  Product1/1 -> Matrix Concatenate/1
  Smtrx/1(S) -> Product1/2
  Ig/1 -> Product2/1
  pqr/1 -> Product2/2, Smtrx/1(a)
  "Smtrx "/1(S) -> Gain1/1
  Transpose/1 -> Product/1
  H/1 -> Product/3, Transpose/1
  Sum/1 -> Product1/1
  " mass (kg) "/1 -> Sum/2  "m"
  mp/1 -> Sum/1  "mp"

== system ROS2_simulink_UE5_0821/Subsystem/Vessel Platform/Input Processing/Inertial Matrix (hull and payload) in CO /Smtrx ==
  a : Inport
  Constant : Constant  Value=0
  Constant1 : Constant  Value=0
  Constant2 : Constant  Value=0
  Create 3x3 Matrix : sharedutil/Create 3x3 Matrix  aMode=aMode
  Demux : Demux  Outputs=3
  Demux1 : Demux  Outputs=3
  Gain : Gain  Gain=-1
  S : Outport
  wires:
  Create 3x3 Matrix/1 -> S/1
  Constant/1 -> Create 3x3 Matrix/1
  a/1 -> Gain/1, Demux/1
  Constant1/1 -> Create 3x3 Matrix/5
  Constant2/1 -> Create 3x3 Matrix/9
  Gain/1 -> Demux1/1
  Demux1/3 -> Create 3x3 Matrix/2
  Demux/2 -> Create 3x3 Matrix/3
  Demux/3 -> Create 3x3 Matrix/4
  Demux1/1 -> Create 3x3 Matrix/6
  Demux1/2 -> Create 3x3 Matrix/7
  Demux/1 -> Create 3x3 Matrix/8

== system ROS2_simulink_UE5_0821/Subsystem/Vessel Platform/Input Processing/Inertial Matrix (hull and payload) in CO /Smtrx1 ==
  a : Inport
  Constant : Constant  Value=0
  Constant1 : Constant  Value=0
  Constant2 : Constant  Value=0
  Create 3x3 Matrix : sharedutil/Create 3x3 Matrix  aMode=aMode
  Demux : Demux  Outputs=3
  Demux1 : Demux  Outputs=3
  Gain : Gain  Gain=-1
  S : Outport
  wires:
  Create 3x3 Matrix/1 -> S/1
  Constant/1 -> Create 3x3 Matrix/1
  a/1 -> Gain/1, Demux/1
  Constant1/1 -> Create 3x3 Matrix/5
  Constant2/1 -> Create 3x3 Matrix/9
  Gain/1 -> Demux1/1
  Demux1/3 -> Create 3x3 Matrix/2
  Demux/2 -> Create 3x3 Matrix/3
  Demux/3 -> Create 3x3 Matrix/4
  Demux1/1 -> Create 3x3 Matrix/6
  Demux1/2 -> Create 3x3 Matrix/7
  Demux/1 -> Create 3x3 Matrix/8

== system ROS2_simulink_UE5_0821/Subsystem/Vessel Platform/Input Processing/Transform CF to CO/Smtrx ==
  a : Inport
  Constant : Constant  Value=0
  Constant1 : Constant  Value=0
  Constant2 : Constant  Value=0
  Create 3x3 Matrix : sharedutil/Create 3x3 Matrix  aMode=aMode
  Demux : Demux  Outputs=3
  Demux1 : Demux  Outputs=3
  Gain : Gain  Gain=-1
  S : Outport
  wires:
  Demux/1 -> Create 3x3 Matrix/8
  Demux1/2 -> Create 3x3 Matrix/7
  Demux1/1 -> Create 3x3 Matrix/6
  Demux/3 -> Create 3x3 Matrix/4
  Demux/2 -> Create 3x3 Matrix/3
  Demux1/3 -> Create 3x3 Matrix/2
  Gain/1 -> Demux1/1
  Constant2/1 -> Create 3x3 Matrix/9
  Constant1/1 -> Create 3x3 Matrix/5
  a/1 -> Demux/1, Gain/1
  Constant/1 -> Create 3x3 Matrix/1
  Create 3x3 Matrix/1 -> S/1

== system ROS2_simulink_UE5_0821/Subsystem/Vessel Platform/Input Processing/Transform CG to CO /Smtrx ==
  a : Inport
  Constant : Constant  Value=0
  Constant1 : Constant  Value=0
  Constant2 : Constant  Value=0
  Create 3x3 Matrix : sharedutil/Create 3x3 Matrix  aMode=aMode
  Demux : Demux  Outputs=3
  Demux1 : Demux  Outputs=3
  Gain : Gain  Gain=-1
  S : Outport
  wires:
  Demux/1 -> Create 3x3 Matrix/8
  Demux1/2 -> Create 3x3 Matrix/7
  Demux1/1 -> Create 3x3 Matrix/6
  Demux/3 -> Create 3x3 Matrix/4
  Demux/2 -> Create 3x3 Matrix/3
  Demux1/3 -> Create 3x3 Matrix/2
  Gain/1 -> Demux1/1
  Constant2/1 -> Create 3x3 Matrix/9
  Constant1/1 -> Create 3x3 Matrix/5
  a/1 -> Demux/1, Gain/1
  Constant/1 -> Create 3x3 Matrix/1
  Create 3x3 Matrix/1 -> S/1

== system ROS2_simulink_UE5_0821/Subsystem/Vessel Platform/Hydrodynamics/Coriolis /Comupute CRB/Smtrx ==
  a : Inport
  Constant : Constant  Value=0
  Constant1 : Constant  Value=0
  Constant2 : Constant  Value=0
  Create 3x3 Matrix : sharedutil/Create 3x3 Matrix  aMode=aMode
  Demux : Demux  Outputs=3
  Demux1 : Demux  Outputs=3
  Gain : Gain  Gain=-1
  S : Outport
  wires:
  Create 3x3 Matrix/1 -> S/1
  Constant/1 -> Create 3x3 Matrix/1
  a/1 -> Gain/1, Demux/1
  Constant1/1 -> Create 3x3 Matrix/5
  Constant2/1 -> Create 3x3 Matrix/9
  Gain/1 -> Demux1/1
  Demux1/3 -> Create 3x3 Matrix/2
  Demux/2 -> Create 3x3 Matrix/3
  Demux/3 -> Create 3x3 Matrix/4
  Demux1/1 -> Create 3x3 Matrix/6
  Demux1/2 -> Create 3x3 Matrix/7
  Demux/1 -> Create 3x3 Matrix/8

== system ROS2_simulink_UE5_0821/Subsystem/Vessel Platform/Hydrodynamics/Coriolis /Comupute CRB/Smtrx  ==
  a : Inport
  Constant : Constant  Value=0
  Constant1 : Constant  Value=0
  Constant2 : Constant  Value=0
  Create 3x3 Matrix : sharedutil/Create 3x3 Matrix  aMode=aMode
  Demux : Demux  Outputs=3
  Demux1 : Demux  Outputs=3
  Gain : Gain  Gain=-1
  S : Outport
  wires:
  Demux/1 -> Create 3x3 Matrix/8
  Demux1/2 -> Create 3x3 Matrix/7
  Demux1/1 -> Create 3x3 Matrix/6
  Demux/3 -> Create 3x3 Matrix/4
  Demux/2 -> Create 3x3 Matrix/3
  Demux1/3 -> Create 3x3 Matrix/2
  Gain/1 -> Demux1/1
  Constant2/1 -> Create 3x3 Matrix/9
  Constant1/1 -> Create 3x3 Matrix/5
  a/1 -> Demux/1, Gain/1
  Constant/1 -> Create 3x3 Matrix/1
  Create 3x3 Matrix/1 -> S/1

== matlab function ROS2_simulink_UE5_0821/simulink2UE5/MATLAB Function1 ==
  data: u1 input; y output; u2 input; u3 input
function y = fcn(u1, u2, u3)
%#codegen
% 将三个标量信号拼成一个 [1x3] 行向量
y = [u1, u2, u3];

== matlab function ROS2_simulink_UE5_0821/simulink2UE5/MATLAB Function ==
  data: u1 input; y output; u2 input; u3 input
function y = fcn(u1, u2, u3)
u1 = u1*5000-9000;
u2 = u2*5000 + 1000;
%#codegen
% 将三个标量信号拼成一个 [1x3] 行向量
y = [u1, u2, u3];

== matlab function ROS2_simulink_UE5_0821/Subsystem/Vessel Platform/Hydrodynamics/Coriolis /Compute CA ==
  data: MA input; CA output; nu_r input
function CA = fcn(MA, nu_r)
% C = m2c(M,nu) computes the Coriolis-centripetal matrix C(nu) from the
% the system inertia matrix M > 0 for varying velocity nu. 
% If M is a 6x6 matrix and nu = [u, v, w, p, q, r]', the output is a 6x6 C matrix
% If M is a 3x3 matrix and nu = [u, v, r]', the output is a 3x3 C matrix.
%
% Examples: CRB = m2c(MRB,nu)     
%           CA  = m2c(MA, nu)
% Output:
%  C         - Coriolis-centripetal matrix C = C(nu) 
%
% Inputs:
%  M        - 6x6 or 3x3 rigid-body MRB or added mass MA system marix 
%  nu       - nu = [u, v, w, p, q, r]' or nu = [u, v, r]'
%
% The Coriolis and centripetal matrix depends on nu1 = [u,v,w]' and nu2 =
% [p,q,r]' as shown in Fossen (2021, Theorem 3.2). It is possible to
% compute C = C(nu2) where nu2 = [p,q,r]' using the linear velocity-
% independent representation, see
%
% [MRB,CRB] = rbody(m,R44,R55,R66,nu2,r_bp) 
%
% Author:    Thor I. Fossen
% Date:      14 Jun 2001
% Revisions: 26 Jun 2002, M21 = M12 is corrected to M12'
%            10 Jan 2004, the computation of C(nU) is generalized to a 
%                         nonsymmetric M > 0 (experimental data)
%            22 Oct 2020, generalized to accept 3-DOF hirizontal-plane models
%            24 Apr 2021, improved the documentation

M = 0.5 * (MA + MA');      % symmetrization of the inertia matrix
nu = nu_r;
    
M11 = M(1:3,1:3);
M12 = M(1:3,4:6);
M21 = M12';
M22 = M(4:6,4:6);

nu1 = nu(1:3);
nu2 = nu(4:6);
dt_dnu1 = M11*nu1 + M12*nu2;
dt_dnu2 = M21*nu1 + M22*nu2;

CA = [  zeros(3,3)      -Smtrx(dt_dnu1)
    -Smtrx(dt_dnu1)  -Smtrx(dt_dnu2) ];


CA(6,1) = 0; % Assume that the Munk moment in yaw can be neglected
CA(6,2) = 0; % These terms, if nonzero, must be balanced by adding nonlinear damping

end

function S = Smtrx(a)
% S = Smtrx(a) computes the 3x3 vector skew-symmetric matrix S(a) = -S(a)'.
% The corss product satisfies: a x b = S(a)b. The inverse can be computed
% as: vex(S(a)) = a 
%
% Author:   Thor I. Fossen
% Date:     14th June 2001
% Revisions: 6th August 2011 - updated documentation
 
S = [    0  -a(3)   a(2)
      a(3)     0   -a(1)
     -a(2)   a(1)     0 ];
end

== matlab function ROS2_simulink_UE5_0821/Subsystem/Vessel Platform/Waves and Crossflow/Compute tau_crossflow ==
  data: L input; B input; T input; tau_crossflow output; nu_r input; rho input
function tau_crossflow = crossFlowDrag(L, B, T, nu_r, rho)

% tau_crossflow = crossFlowDrag(L,B,T,nu_r) computes the cross-flow drag 
% integrals for a marine craft using strip theory. Application:
%
%  M d/dt nu_r + C(nu_r)*nu_r + D*nu_r + g(eta) = tau + tau_crossflow
%
% Inputs: L:  length
%         B:  beam
%         T:  draft 
%         nu_r = [u-u_c, v-v_c, w-w_c, p, q, r]': relative velocity vector
%
% Output: tau_crossflow = [0 Yh 0 0 0 Nh]:  cross-flow drag in sway and yaw
%
% Author:     Thor I. Fossen 
% Date:       25 Apr 2021
% Revisions:  

% rho = 1026;             % density of water
n = 20;                 % number of strips

dx = L/20;             
Cd_2D = Hoerner(B,T);   % 2D drag coefficient based on Hoerner's curve

Yh = 0;
Nh = 0;
for xL = -L/2:dx:L/2
    v_r = nu_r(2);          % relative sway velocity
    r = nu_r(6);            % yaw rate
    Ucf = abs(v_r + xL * r) * (v_r + xL * r);
    Yh = Yh - 0.5 * rho * T * Cd_2D * Ucf * dx;         % sway force
    Nh = Nh - 0.5 * rho * T * Cd_2D * xL * Ucf * dx;    % yaw moment
end

tau_crossflow = [0 Yh 0 0 0 Nh]';

end

function CY_2D = Hoerner(B,T)
% Hoerner computes the 2D Hoerner cross-flow form coeff. as a function of B and T.
% he data is digizied and interpolation is used to compute other data points 
% than those in the table
%
%  CY_2D = Hoerner(B,T)
%
% Output: 
%    CY_2D:    2D Hoerner cross-flow form coefficient
%
% Inputs:
%    T:      draft (m)
%    B:      beam  (m)
%
% Author: Thor I. Fossen
% Date:   2007-12-01
%
% Reference:
% A. J. P. Leite, J. A. P. Aranha, C. Umeda and M. B. conti (1998). 
% Current force in tankers and bifurcation of equilibrium of turret
% systems: hydrodynamic model and experiments. 
% Applied Ocean Research 20, pp. 145-256.

% CD_DATA = [B/2T  C_D]
CD_DATA = [...    
0.0108623 1.96608
0.176606 1.96573
0.353025 1.89756
0.451863 1.78718
0.472838 1.58374
0.492877 1.27862
0.493252 1.21082
0.558473 1.08356
0.646401 0.998631
0.833589 0.87959
0.988002 0.828415
1.30807 0.759941
1.63918 0.691442
1.85998 0.657076
2.31288 0.630693
2.59998 0.596186
3.00877 0.586846
3.45075 0.585909
3.7379 0.559877
4.00309 0.559315];

CY_2D = interp1(CD_DATA(:,1),CD_DATA(:,2),B/(2*T));
end

== matlab function ROS2_simulink_UE5_0821/simulink2UE1/MATLAB Function ==
  data: u1 input; y output; u2 input; u3 input
function y = fcn(u1, u2, u3)
u1 = u1*100+32660; % unit in UE5: cm
u2 = u2*100 - 13050;
%#codegen
% 将三个标量信号拼成一个 [1x3] 行向量
y = [u1, u2, u3];

== matlab function ROS2_simulink_UE5_0821/simulink2UE1/MATLAB Function1 ==
  data: u1 input; y output; u2 input; u3 input
function y = fcn(u1, u2, u3)
%#codegen
% 将三个标量信号拼成一个 [1x3] 行向量
y = [u1, u2, u3];

== matlab function ROS2_simulink_UE5_0821/Subsystem/Vessel Platform/Thrust/MATLAB Function ==
  data: n_sig input; T_N output
function T_N = rpm2thrust(n_sig)
% n_sig: 转速信号 (rpm 向量或标量都可以)
% 输出: 推力 (N)，与输入维度一致

A = 8.18448e-05;   % kN / rpm^q
q = 2.17020;

% 如输入是 rad/s，请把下一行打开；如本来就是 rpm，则保持注释
% n_sig = n_sig * 60/(2*pi);  % rad/s -> rpm

% 幂律关系
TkN = sign(n_sig) .* (abs(n_sig).^q) * A;   % 单位: kN
T_N = 1000 * TkN;                           % 转换为 N

% -------- 低速死区处理 (逐元素) --------
% 建立逻辑索引，找到绝对值小于阈值的元素
idx = abs(n_sig) < 1e-3;
T_N(idx) = 0;
